simulink model "Masse_Feder_Fluid_model"  (R2024a)
settings: Solver=FixedStepAuto  StartTime=0.0  StopTime=100  FixedStep=0.01  RelTol=1e-3
values from neighbouring files (symbols this model uses):
  b = 100e3    (= 100000)    [Masse_Feder_Fluid_param.m]
  k = 100    [Masse_Feder_Fluid_param.m]
  m = 10    [Masse_Feder_Fluid_param.m]
settings Model: Creator=fldr  LastModifiedBy=fldr

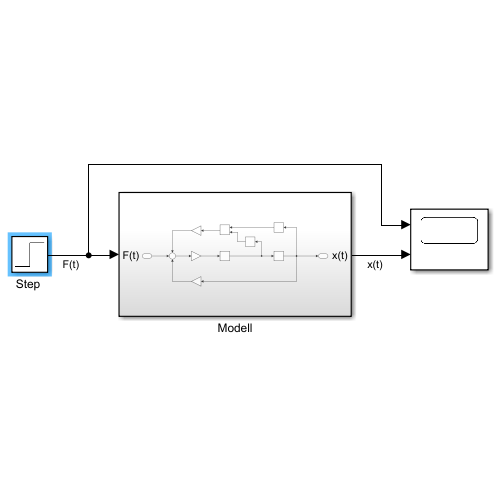
[thumbnail: Simulink's stored preview of the top-level diagram]
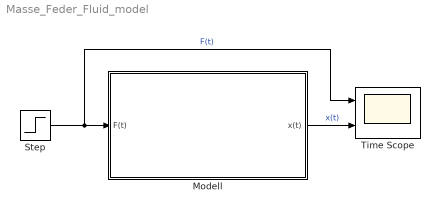
== system Masse_Feder_Fluid_model ==
  Modell : Subsystem
  "Step " : Step  Time=10  SampleTime=0
  Time Scope : Scope  NumInputPorts=2
      settings: CopyFcn=try ZHAWcbfcn('copyScope'); end  NameChangeFcn=try ZHAWcbfcn('namechangeScope'); end
  wires:
  "Step "/1 -> Time Scope/1, Modell/1(F(t))  "F(t)"
  Modell/1(x(t)) -> Time Scope/2  "x(t)"

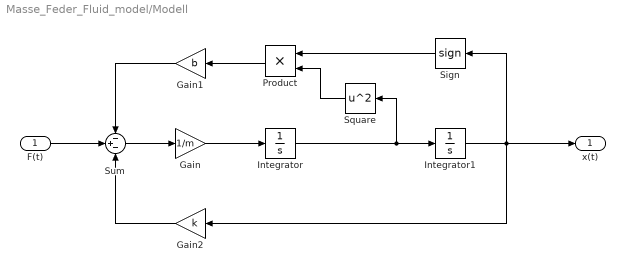
== system Masse_Feder_Fluid_model/Modell ==
  F(t) : Inport
  Gain : Gain  Gain=1/m
  Gain1 : Gain  Gain=b
  Gain2 : Gain  Gain=k
  Integrator : Integrator
  Integrator1 : Integrator
  Product : Product
  Sign : Signum
  Square : Math  Operator=square
  Sum : Sum  Inputs=-+-
  x(t) : Outport
  wires:
  Gain2/1 -> Sum/3
  Integrator/1 -> Square/1, Integrator1/1
  Sign/1 -> Product/1
  F(t)/1 -> Sum/2
  Integrator1/1 -> x(t)/1, Gain2/1, Sign/1
  Product/1 -> Gain1/1
  Square/1 -> Product/2
  Gain1/1 -> Sum/1
  Sum/1 -> Gain/1
  Gain/1 -> Integrator/1
